simulink model "TL2K_VL10_model"  (R2017a)
settings: Solver=FixedStepDiscrete  StartTime=0.0  StopTime=0.1  FixedStep=1e-4  RelTol=1e-3
values from neighbouring files (symbols this model uses):
  A = 1570    [TractionCharacteristic.m]
  B = 6.3    [TractionCharacteristic.m]
undefined symbols (not defined in the file or in its folder): modelLocomotiveSpeed
libraries: powerlib x2, eltreclib x2
settings Model: Creator=mayartmal  LastModifiedBy=mayartmal
settings SolverCC: AlgebraicLoopSolver=LineSearch

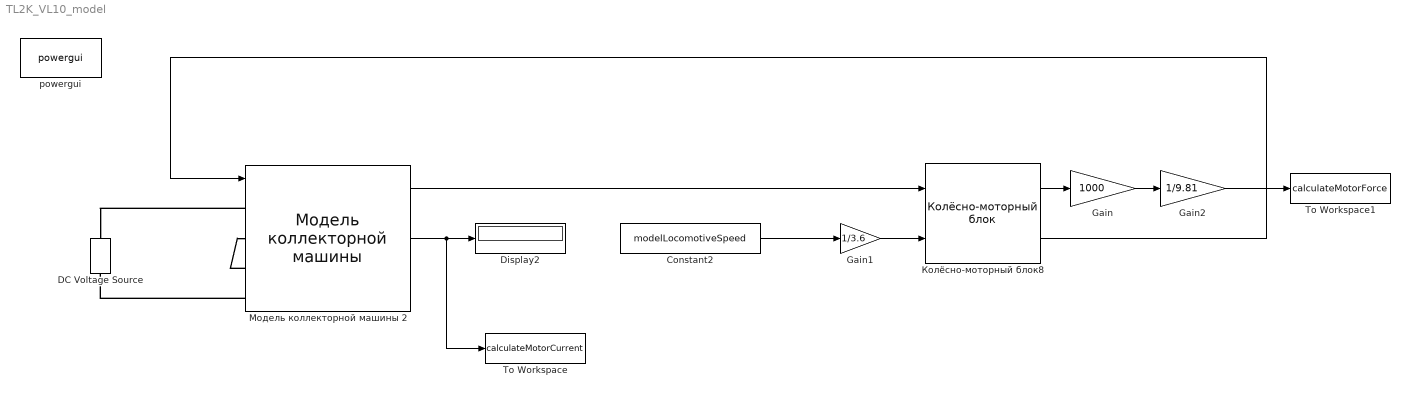
== system TL2K_VL10_model ==
  Constant2 : Constant  Value=modelLocomotiveSpeed
  DC Voltage Source : powerlib/Electrical Sources/DC Voltage Source  Amplitude=1500  Measurements=None
  Display2 : Display
  Gain : Gain  Gain=1000
  Gain1 : Gain  Gain=1/3.6
  Gain2 : Gain  Gain=1/9.81
  To Workspace : ToWorkspace  VariableName=calculateMotorCurrent  SampleTime=-1
      settings: MaxDataPoints=1
  To Workspace1 : ToWorkspace  VariableName=calculateMotorForce  SampleTime=-1
      settings: MaxDataPoints=1
  powergui : powerlib/powergui  Priority=1  SimulationMode=Discrete  SampleTime=1e-4  frequency=60  Iterations=50  frequencyindice=0  Pbase=100e6  ErrMax=1e-4  UnitsV=kV  UnitsW=MW  buscounter=0  FunctionMessages=off  echomessages=off  EnableUseOfTLC=off  CurrentSourceSwitches=off  DisableSnubberDevices=off  DisableRonSwitches=off  DisableVfSwitches=off  DisplayEquations=off  SolverType=Tustin/Backward Euler (TBE)  Interpol=off  ExternalGateDelay=off  methode=off  Ts=100  x0status=blocks  SPID=on  SwTol=0  HookPort=off  RestoreLinks=warning  ResistiveCurrentMeasurement=off  Frange=[0:2:500]  Ylog=off  Xlog=on  ShowGrid=off  save=off  variable=ZData  structure=0  ZoomFFT=off  StartTime=0.0  cycles=1  DisplayStyle=1  fundamental=60  FreqAxis=off  MaxFrequency=1000  frequencyindicesteady=1  RmsSteady=1  display=off
  Колёсно-моторный блок8 : eltreclib/Колёсно-моторный блок  Db=1.25  mu=3.826
      settings: SourceProductName=Electric Traction
  Модель коллекторной машины 2 : eltreclib/Модель коллекторной машины  Rf=0.036  Lf=0.0002  Ra=0.0673  La=0.005  Ce=167.113  Cm=167.113  A=A  B=B
      settings: SourceProductName=Electric Traction
  wires:
  Модель коллекторной машины 2/1 -> Колёсно-моторный блок8/1
  Модель коллекторной машины 2/2 -> To Workspace/1, Display2/1
  Constant2/1 -> Gain1/1
  Колёсно-моторный блок8/2 -> Модель коллекторной машины 2/1
  Gain1/1 -> Колёсно-моторный блок8/2
  Колёсно-моторный блок8/1 -> Gain/1
  Gain/1 -> Gain2/1
  Gain2/1 -> To Workspace1/1
  connections:
  Модель коллекторной машины 2/LConn1 -- DC Voltage Source/RConn1
  Модель коллекторной машины 2/LConn4 -- DC Voltage Source/LConn1
  Модель коллекторной машины 2/LConn3 -- Модель коллекторной машины 2/LConn2
